simulink model "lab4complex"  (Simulink 7.7)
settings: Solver=ode45  StartTime=0.0  StopTime=10.0  RelTol=1e-3
libraries: cstblocks x7
settings Model: Creator=Muhammad Ali khan  LastModifiedBy=Muhammad Ali khan

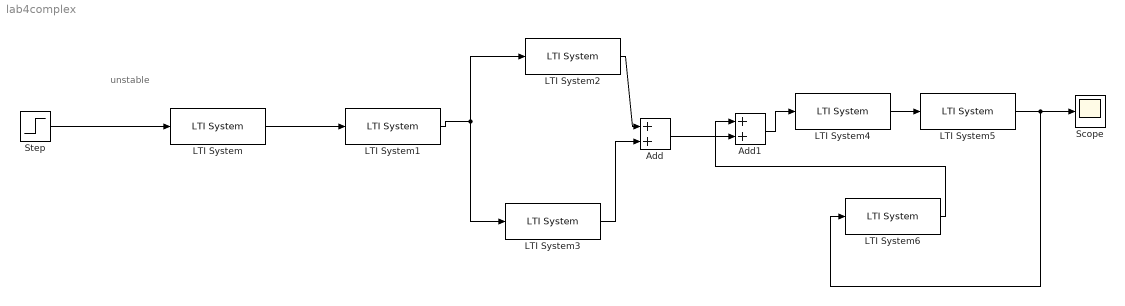
== system lab4complex ==
  note: unstable
  Add : Sum
  Add1 : Sum
  LTI System : cstblocks/LTI System  SystemSampleTime=-1  sys=tf([1 ],[1 1])  IC=[]
  LTI System1 : cstblocks/LTI System  SystemSampleTime=-1  sys=tf([1],[1 3])  IC=[]
  LTI System2 : cstblocks/LTI System  SystemSampleTime=-1  sys=tf([1 3],[1 5])  IC=[]
  LTI System3 : cstblocks/LTI System  SystemSampleTime=-1  sys=tf([1 ],[1 1])  IC=[]
  LTI System4 : cstblocks/LTI System  SystemSampleTime=-1  sys=tf([1],[1 3])  IC=[]
  LTI System5 : cstblocks/LTI System  SystemSampleTime=-1  sys=tf([1 3],[1 5])  IC=[]
  LTI System6 : cstblocks/LTI System  SystemSampleTime=-1  sys=tf([1 3],[1 5])  IC=[]
  Scope : Scope
  Step : Step  SampleTime=0
  wires:
  Step/1 -> LTI System/1
  LTI System/1 -> LTI System1/1
  LTI System4/1 -> LTI System5/1
  LTI System5/1 -> Scope/1, LTI System6/1
  LTI System2/1 -> Add/1
  LTI System3/1 -> Add/2
  Add/1 -> Add1/2
  Add1/1 -> LTI System4/1
  LTI System1/1 -> LTI System2/1, LTI System3/1
  LTI System6/1 -> Add1/1
